simulink model "bondarkoLastTask"  (R2018a)
settings: Solver=VariableStepAuto  StartTime=0.0  StopTime=300  RelTol=1e-3
libraries: dspsrcs4 x1
settings Model: Creator=Петр  LastModifiedBy=Петр

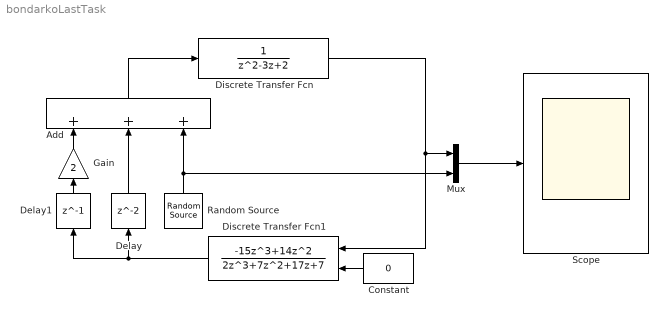
== system bondarkoLastTask ==
  Add : Sum  Inputs=+++
  Constant : Constant  Value=0
  Delay : Delay  SampleTime=0.1
  Delay1 : Delay  DelayLength=1
  Discrete Transfer Fcn : DiscreteTransferFcn  Denominator=[1 -3 2]  SampleTime=0.1
  Discrete Transfer Fcn1 : DiscreteTransferFcn  Numerator=[-15 14 0 0]  Denominator=[2 7 17 7]  InitialStatesSource=Input port  InitialStates=4  SampleTime=0.1
      settings: InputPortMap=u0,p5
  Gain : Gain  Gain=2
  Mux : Mux  Inputs=2
  Random Source : dspsrcs4/Random Source  SrcType=Uniform  NormMethod=Ziggurat  CltLength=12  MinVal=-1  MaxVal=1  MeanVal=0  VarVal=1  RepMode=Not repeatable  rawSeed=1  IsInherit=off  SampMode=Discrete  SampTime=1  SampFrame=1  DataType=Double  OutComplex=Real  OutputFrames=off
  Scope : Scope
  wires:
  Discrete Transfer Fcn1/1 -> Delay1/1, Delay/1
  Add/1 -> Discrete Transfer Fcn/1
  Discrete Transfer Fcn/1 -> Mux/1, Discrete Transfer Fcn1/1
  Constant/1 -> Discrete Transfer Fcn1/2
  Delay/1 -> Add/2
  Gain/1 -> Add/1
  Delay1/1 -> Gain/1
  Random Source/1 -> Add/3, Mux/2
  Mux/1 -> Scope/1
